simulink model "Control1_BA"  (R2023b)
settings: Solver=FixedStepAuto  StartTime=0.0  StopTime=inf  RelTol=1e-3  EnableMultiTasking=on
settings Model: ExtModeTrigDuration=2  Creator=Usuario  LastModifiedBy=Usuario
settings OptimizationCC: EnhancedBackFolding=on  PassReuseOutputArgsAs=Individual arguments  ZeroExternalMemoryAtStartup=off  ZeroInternalMemoryAtStartup=off  MaxStackSize=64  OptimizeBlockOrder=speed  DifferentSizesBufferReuse=on  OptimizationCustomize=off  EfficientTunableParamExpr=on
settings DebuggingCC: ParameterTunabilityLossMsg=error
settings HardwareCC: ProdBitPerInt=16  ProdBitPerPointer=16  ProdBitPerSizeT=16  ProdBitPerPtrDiffT=16  ProdLargestAtomicFloat=None  ProdWordSize=8  ProdHWDeviceType=Atmel->AVR  UseEmbeddedCoderFeatures=off  UseSimulinkCoderFeatures=off
settings SFSimCC: MATLABDynamicMemAlloc=off
settings RTWCC: Description=Embedded Coder  SystemTargetFile=ert.tlc  HardwareBoard=Arduino Mega 2560  TemplateMakefile=ert_default_tmf  Toolchain=Arduino AVR  BuildConfiguration=Faster Runs
settings CodeAppCC: ForceParamTrailComments=on  IgnoreCustomStorageClasses=off  OperatorAnnotations=on  SimulinkDataObjDesc=on  SFDataObjDesc=on  InsertBlockDesc=on
settings ERTTargetCC: SupportContinuousTime=on  SupportNonInlinedSFcns=on  SupportVariableSizeSignals=on  ExtModeTransport=3  ExtModeStaticAlloc=on  ExtModeAutomaticAllocSize=off  ExtModeStaticAllocSize=2048  ExtModeMexFile=ext_xcp  ExtModeIntrfLevel=Level2 - Open

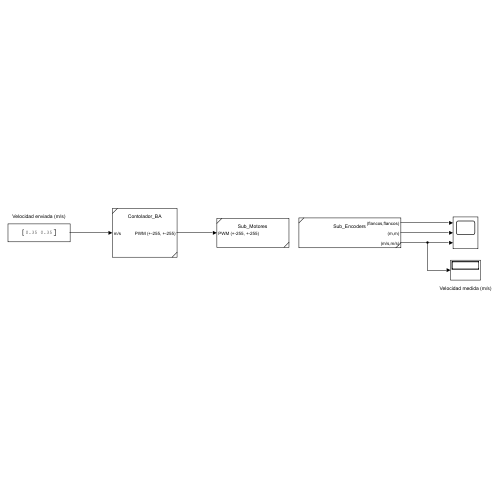
[thumbnail: Simulink's stored preview of the top-level diagram]
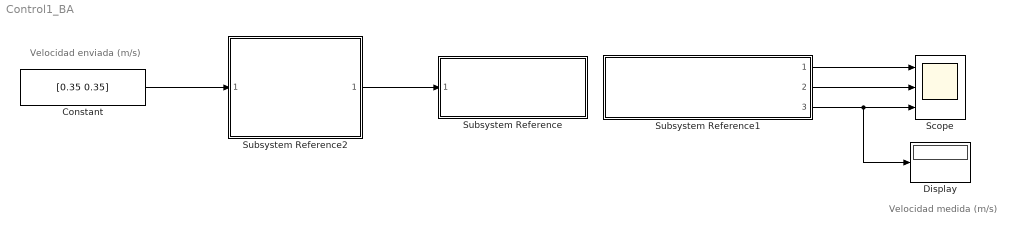
== system Control1_BA ==
  note: Velocidad medida (m/s)
  note: Velocidad enviada (m/s)
  Constant : Constant  Value=[0.35 0.35]
  Display : Display
  Scope : Scope  NumInputPorts=3
  Subsystem Reference : Subsystem  ReferencedSubsystem=Sub_Motores
  Subsystem Reference1 : Subsystem  ReferencedSubsystem=Sub_Encoders
  Subsystem Reference2 : Subsystem  ReferencedSubsystem=Contolador_BA
  wires:
  Subsystem Reference1/1 -> Scope/1
  Subsystem Reference1/2 -> Scope/2
  Subsystem Reference1/3 -> Display/1, Scope/3
  Constant/1 -> Subsystem Reference2/1
  Subsystem Reference2/1 -> Subsystem Reference/1
